simulink model "GPS_pll"  (Simulink 6.1)
settings: Solver=ode45  StartTime=0.0  StopTime=5000  RelTol=1e-5
values from neighbouring files (symbols this model uses):
  Ga = 2    [GPS_pll_init.m]    (also in GPS_pll_init_148.m = 0.0625; GPS_pll_init_bak.m = 0.03125)
  Gb = 2    [GPS_pll_init.m]    (also in GPS_pll_init_148.m = 16; GPS_pll_init_bak.m)
  Gdac = 2^-16*5    (= 7.62939453125e-05)    [GPS_pll_init.m]    (also in GPS_pll_init_148.m; GPS_pll_init_bak.m = 5.03540039062e-05)
  Kv = 4e-6    (= 4e-06)    [GPS_pll_init.m]    (also in GPS_pll_init_148.m = 9e-05; GPS_pll_init_bak.m)
  Ts = 1/100e6    (= 1e-08)    [GPS_pll_init.m]    (also in GPS_pll_init_148.m = 6.73400673401e-09; GPS_pll_init_bak.m = 5e-09)
libraries: simulink x1
settings Model: LastModifiedBy=jkh
settings DataIOCC: SignalLoggingName=sigsOut
settings HardwareCC: TargetUnknown=on

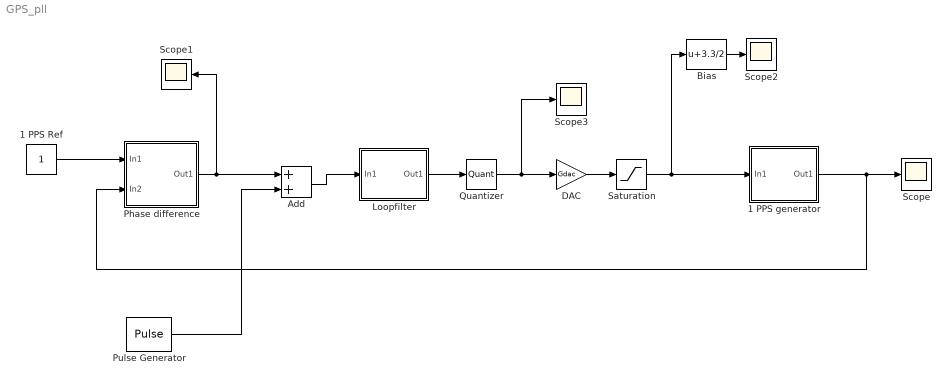
== system GPS_pll ==
  1 PPS Ref : Constant
  1 PPS generator : Subsystem
  Add : Sum  OutScaling=2^-10
  Bias : Bias  Bias=3.3/2
  DAC : Gain  Gain=Gdac  SaturateOnIntegerOverflow=on
  Loopfilter : Subsystem
  Phase difference : Subsystem
  Pulse Generator : DiscretePulseGenerator  PulseType=Time based  Amplitude=512  Period=1000  PulseWidth=50
  Quantizer : Quantizer  QuantizationInterval=1
  Saturation : Saturate  UpperLimit=3.3/2  LowerLimit=-3.3/2
  Scope{,1..3} (4 alike) : Scope
      Scope1 settings: SampleInput=on  SampleTime=1
      Scope2 settings: TimeRange=5.22433885907202  YMin=1.62  YMax=1.74  SaveName=ScopeData2  SampleInput=on  SampleTime=1
      Scope3 settings: SaveName=ScopeData3  SampleInput=on  SampleTime=1
  wires:
  1 PPS Ref/1 -> Phase difference/1(In1)
  1 PPS generator/1(Out1) -> Scope/1, Phase difference/2(In2)
  Phase difference/1(Out1) -> Scope1/1, Add/1
  DAC/1 -> Saturation/1
  Quantizer/1 -> DAC/1, Scope3/1
  Saturation/1 -> 1 PPS generator/1(In1), Bias/1
  Loopfilter/1(Out1) -> Quantizer/1
  Add/1 -> Loopfilter/1(In1)
  Pulse Generator/1 -> Add/2
  Bias/1 -> Scope2/1

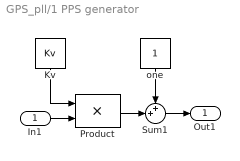
== system GPS_pll/1 PPS generator ==
  In1 : Inport  Port=1  LatchInput=off
  Kv : Constant  Orientation=down  Value=Kv
  Product : Product  SaturateOnIntegerOverflow=on
  Sum1 : Sum  Inputs=++|  SaturateOnIntegerOverflow=on
  one : Constant  Orientation=down
  Out1 : Outport
  wires:
  Kv/1 -> Product/1
  Product/1 -> Sum1/2
  one/1 -> Sum1/1
  Sum1/1 -> Out1/1
  In1/1 -> Product/2

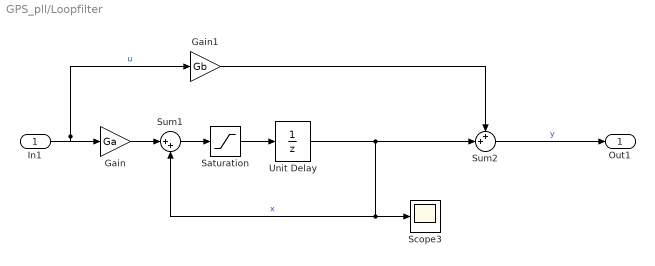
== system GPS_pll/Loopfilter ==
  In1 : Inport  Port=1  LatchInput=off
  Gain : Gain  Gain=Ga  SaturateOnIntegerOverflow=on
  Gain1 : Gain  Gain=Gb  SaturateOnIntegerOverflow=on
  Saturation : Saturate  UpperLimit=2^15*(3.3/5)  LowerLimit=-2^15*(3.3/5)
  Scope3 : Scope
      settings: SaveName=ScopeData4  SampleInput=on  SampleTime=1
  Sum1 : Sum  Inputs=|++  SaturateOnIntegerOverflow=on
  Sum2 : Sum  Inputs=++|  SaturateOnIntegerOverflow=on
  Unit Delay : UnitDelay
  Out1 : Outport
  wires:
  In1/1 -> Gain1/1, Gain/1  "u"
  Gain1/1 -> Sum2/1
  Sum2/1 -> Out1/1  "y"
  Gain/1 -> Sum1/1
  Sum1/1 -> Saturation/1
  Saturation/1 -> Unit Delay/1
  Unit Delay/1 -> Sum2/2, Sum1/2, Scope3/1  "x"

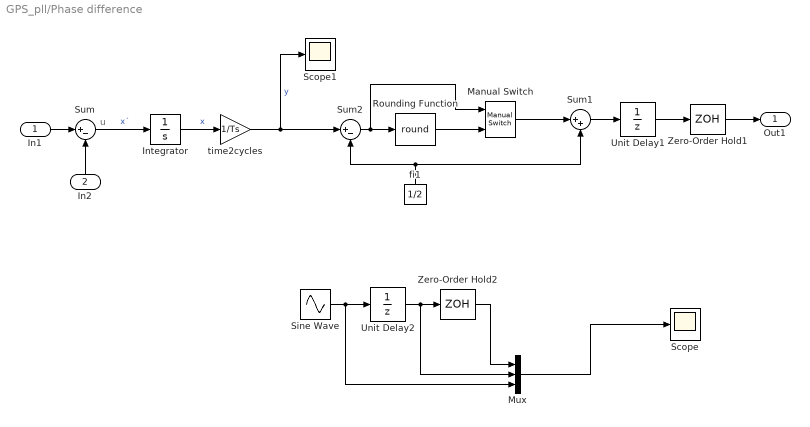
== system GPS_pll/Phase difference ==
  note: u
  In1 : Inport  Port=1  LatchInput=off
  In2 : Inport  Orientation=up  Port=2  LatchInput=off
  Integrator : Integrator  InitialCondition=7000*Ts
  Manual Switch : simulink/Signal Routing/Manual Switch  sw=0  action=0
  Mux : Mux  Inputs=3
  Rounding Function : Rounding  Operator=round
  Scope : Scope
      settings: SaveName=ScopeData6  SampleInput=on
  Scope1 : Scope
      settings: SaveName=ScopeData5  SampleInput=on  SampleTime=1
  Sine Wave : Sin  SampleTime=0
  Sum : Sum  Inputs=|+-  SaturateOnIntegerOverflow=on
  Sum1 : Sum  Inputs=|++  SaturateOnIntegerOverflow=on
  Sum2 : Sum  Inputs=|+-  SaturateOnIntegerOverflow=on
  Unit Delay1 : UnitDelay  SampleTime=0.5
  Unit Delay2 : UnitDelay  SampleTime=0.5
  Zero-Order Hold1 : ZeroOrderHold
  Zero-Order Hold2 : ZeroOrderHold
  fi1 : Constant  Orientation=up  Value=1/2
  time2cycles : Gain  Gain=1/Ts  SaturateOnIntegerOverflow=on
  Out1 : Outport
  wires:
  Sum/1 -> Integrator/1  "x´"
  In2/1 -> Sum/2
  Integrator/1 -> time2cycles/1  "x"
  In1/1 -> Sum/1
  fi1/1 -> Sum1/2, Sum2/2
  Sum2/1 -> Manual Switch/1, Rounding Function/1
  Sum1/1 -> Unit Delay1/1
  Manual Switch/1 -> Sum1/1
  Rounding Function/1 -> Manual Switch/2
  time2cycles/1 -> Sum2/1, Scope1/1  "y"
  Unit Delay1/1 -> Zero-Order Hold1/1
  Zero-Order Hold1/1 -> Out1/1
  Unit Delay2/1 -> Zero-Order Hold2/1, Mux/2
  Sine Wave/1 -> Unit Delay2/1, Mux/3
  Zero-Order Hold2/1 -> Mux/1
  Mux/1 -> Scope/1
